simulink model "FiveHundredmeterpossible"  (R2020b)
settings: Solver=ode5  StartTime=0.0  StopTime=600  FixedStep=0.001  RelTol=1e-3
model workspace (MATLAB code in the model file):
  | P=10000
  | I=1000
  | D=10000
  | k=2%set [1, 2, 4] to choose the battery
  | r = 0.1 %halfradious of the wheel
  | J = (0.5*r)*r*r  %inertia of wheel
  | V=12*k %voltage of the battery
  | mm= 0.34 %motor mass
  | bm= 0.1*k %battery mass
  | Kt= 29.2*10^(-3) %75.6*10^(-3) %motor thingy
  | Ke= 1/328%1/126 %motor thingy
  | R= 0.582 %motor resistence
  | b=0 %friction
  | K=Kt/(b*R+Kt*Ke)
  | T=(R*J)/(b*R+Kt*Ke)
  | 
  | a=(r*r*R)/(10*Kt)
  | b=5*Ke/r
undefined symbols (not defined in the file): M
libraries: eePwmGenerator x1
settings Model: OrderedModelArguments=off  Creator=melih.turkseven  LastModifiedBy=Erkin
settings SolverCC: ZeroCrossAlgorithm=Adaptive
settings DebuggingCC: IgnoredZcDiagnostic=none
settings SFSimCC: CustomCodeUndefinedFunction=UseInterfaceOnly

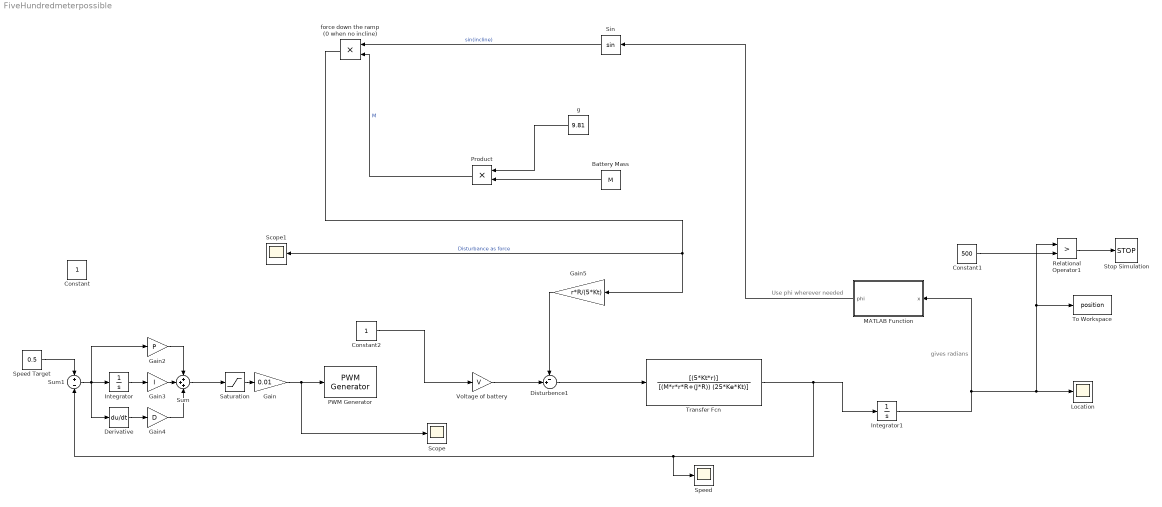
== system FiveHundredmeterpossible ==
  note: gives radians
  note: Use phi wherever needed
  Battery Mass : Constant  Value=M
  Constant1 : Constant  Value=500
  Constant2 : Constant
  Derivative : Derivative
  Disturbence1 : Sum  Inputs=-+|
  Gain : Gain  Gain=0.01
  Gain2 : Gain  Gain=P
  Gain3 : Gain  Gain=I
  Gain4 : Gain  Gain=D
  Gain5 : Gain  Gain=r*R/(5*Kt)
  Integrator : Integrator
  Integrator1 : Integrator
  Location : Scope
  MATLAB Function : MATLAB Function  TreatAsAtomicUnit=on
  PWM Generator : eePwmGenerator/PWM Generator  CarrCount=Up  Tper=0.01  Ts=0.001
  Product : Product
  Relational Operator1 : RelationalOperator  Operator=>  OutDataTypeStr=boolean  RndMeth=Simplest
  Saturation : Saturate  UpperLimit=100  LowerLimit=0
  Scope : Scope
  Scope1 : Scope
  Sin : Trigonometry
  Speed : Scope
  Speed Target : Constant  Value=0.5
  Stop Simulation : Stop
  Sum : Sum  Inputs=+++
  Sum1 : Sum  Inputs=+-
  To Workspace : ToWorkspace  VariableName=position  SampleTime=-1
  Transfer Fcn : TransferFcn  Numerator=[(5*Kt*r)]  Denominator=[(M*r*r*R+(J*R)) (25*Ke*Kt)]
  Voltage of battery : Gain  Gain=V
  force down the ramp (0 when no incline) : Product
  g : Constant  Value=9.81
  Constant : Constant  IOType=siggen
  wires:
  Relational Operator1/1 -> Stop Simulation/1
  Gain/1 -> Scope/1, PWM Generator/1
  Saturation/1 -> Gain/1
  Sum/1 -> Saturation/1
  Gain3/1 -> Sum/2
  Gain2/1 -> Sum/1
  Gain4/1 -> Sum/3
  Integrator/1 -> Gain3/1
  Derivative/1 -> Gain4/1
  Constant1/1 -> Relational Operator1/2
  Sum1/1 -> Gain2/1, Derivative/1, Integrator/1
  g/1 -> Product/1
  Product/1 -> force down the ramp (0 when no incline)/2  "M"
  Sin/1 -> force down the ramp (0 when no incline)/1  "sin(incline)"
  MATLAB Function/1(phi) -> Sin/1
  Speed Target/1 -> Sum1/1
  force down the ramp (0 when no incline)/1 -> Gain5/1, Scope1/1  "Disturbance as force"
  Voltage of battery/1 -> Disturbence1/2
  Gain5/1 -> Disturbence1/1
  Disturbence1/1 -> Transfer Fcn/1
  Battery Mass/1 -> Product/2
  Transfer Fcn/1 -> Speed/1, Sum1/2, Integrator1/1
  Constant2/1 -> Voltage of battery/1
  Integrator1/1 -> Location/1, Relational Operator1/1, To Workspace/1, MATLAB Function/1(x)

== matlab function FiveHundredmeterpossible/MATLAB Function ==
  data: x input; phi output
function phi = getInclination(x)

if x < 250
    phi = 0;
else
    if x < 350
        phi = pi / 6;
    else
        phi = pi / 18;
    end
end
